simulink model "rrcrov2_para"  (Simulink 6.0)
settings: Solver=ode4  StartTime=0.0  StopTime=0.1  FixedStep=0.1  MaxStep=0.1  RelTol=0.5
undefined symbols (not defined in the file): B, DQ, DQL, M, Ma, rg, T, W, zb, zg
settings Model: LastModifiedBy=c

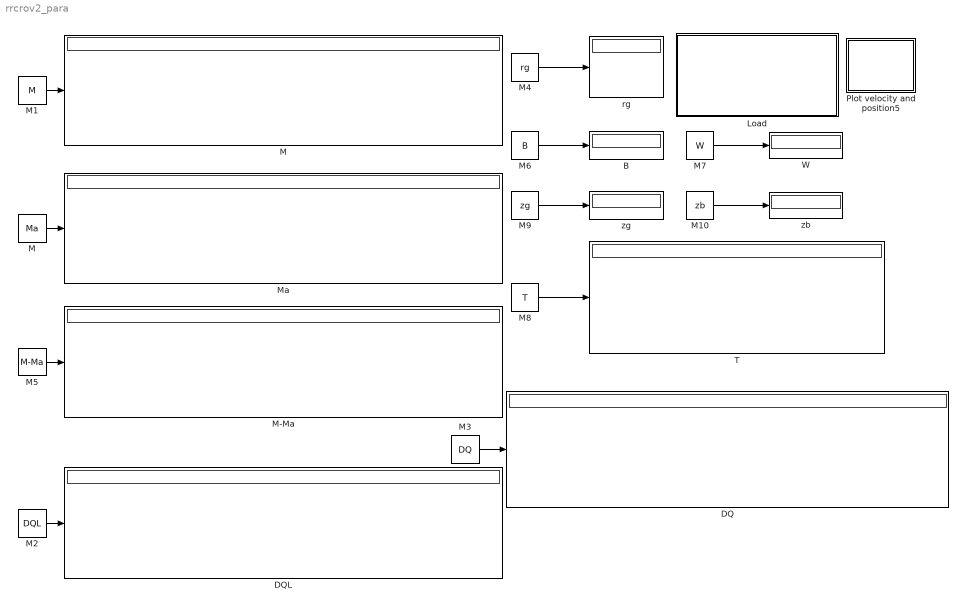
== system rrcrov2_para ==
  " Load  " : Subsystem  AncestorBlock=|
      | rov_design_analysis/ROV Controller
      | Design
      | Applications/ Load RRCROV2 parameters
      settings: OpenFcn=|
      | clc
      | cd c:\Matlab7\toolbox\rov_design_analysis\\mat_file ;
      | load rrcrovf;
      mask Display: disp('Double-click \n to \n Load the\n RRCROV\n parameters')
  B : Display
  "DQ " : Display
  DQL : Display
  M : Constant  Value=Ma
  "M   " : Display
  M-Ma : Display
  M1 : Constant  Value=M
  M10 : Constant  Value=zb
  M2 : Constant  Value=DQL
  M3 : Constant  Value=DQ
  M4 : Constant  Value=rg
  M5 : Constant  Value=M-Ma
  M6 : Constant  Value=B
  M7 : Constant  Value=W
  M8 : Constant  Value=T
  M9 : Constant  Value=zg
  Ma : Display
  Plot velocity and position5 : Subsystem  AncestorBlock=|
      | rov_design_analysis/ROV Controller
      | Design
      | Applications/Plot velocity and position
      settings: OpenFcn=|
      | clc
      | cd c:\Matlab7\toolbox\rov_design_analysis\hybrid
      | sim('rrcrov2_para')
      mask Display: disp('Show')
  T : Display
  W : Display
  rg : Display
  zb : Display
  zg : Display
  wires:
  M1/1 -> "M   "/1
  M/1 -> Ma/1
  M5/1 -> M-Ma/1
  M2/1 -> DQL/1
  M3/1 -> "DQ "/1
  M4/1 -> rg/1
  M6/1 -> B/1
  M7/1 -> W/1
  M8/1 -> T/1
  M9/1 -> zg/1
  M10/1 -> zb/1

== system rrcrov2_para/ Load   ==

== system rrcrov2_para/Plot velocity and position5 ==
